simulink model "speedconversion"  (R2016a)
settings: Solver=VariableStepAuto  SolverMode=SingleTasking  StartTime=0.0  StopTime=10.0  RelTol=1e-3
settings Model: Creator=karanverma  LastModifiedBy=karanverma
settings DebuggingCC: SFUnexpectedBacktrackingDiag=error  SFNoUnconditionalDefaultTransitionDiag=error
settings GRTTargetCC: TargetLangStandard=C99 (ISO)  GeneratePreprocessorConditionals=Use local settings
settings ConfigComp: CovMetricSettings=dwe  CovHtmlReporting=off  CovSaveCumulativeToWorkspaceVar=off  CovSaveSingleToWorkspaceVar=off  CovExternalEMLEnable=on

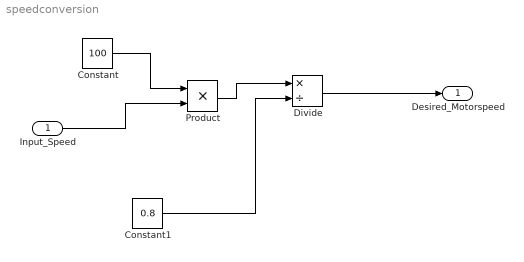
== system speedconversion ==
  Input_Speed : Inport
  Constant : Constant  Value=100
  Constant1 : Constant  Value=0.8
  Divide : Product  Inputs=*/
  Product : Product
  Desired_Motorspeed : Outport
  wires:
  Input_Speed/1 -> Product/2
  Constant/1 -> Product/1
  Constant1/1 -> Divide/2
  Product/1 -> Divide/1
  Divide/1 -> Desired_Motorspeed/1
